simulink model "OpenLoopResponse"  (R2016a)
settings: Solver=VariableStepAuto  StartTime=0.0  StopTime=30  MaxStep=.005  RelTol=1e-3
libraries: simulink x1
settings Model: Creator=jordan  LastModifiedBy=jordan

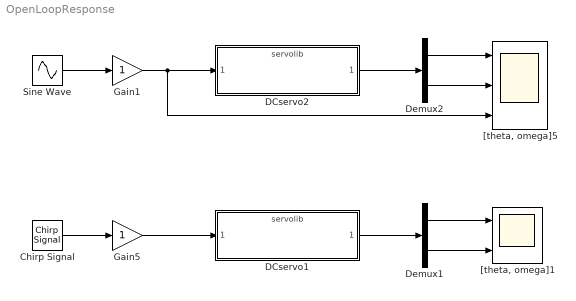
== system OpenLoopResponse ==
  Chirp Signal : simulink/Sources/Chirp Signal  f1=.01  T=120  f2=10
  DCservo1 : ModelReference  ModelNameDialog=servolib.slx  SimulationMode=Normal  ModelReferenceVersion=1.68
  DCservo2 : ModelReference  ModelNameDialog=servolib.slx  SimulationMode=Normal  ModelReferenceVersion=1.68
  Demux1 : Demux  Outputs=2
  Demux2 : Demux  Outputs=2
  Gain1 : Gain
  Gain5 : Gain
  Sine Wave : Sin  Frequency=10  SampleTime=0
  "[theta, omega]1" : Scope  NumInputPorts=2
  "[theta, omega]5" : Scope  NumInputPorts=3
  wires:
  DCservo2/1 -> Demux2/1
  Demux2/2 -> "[theta, omega]5"/2
  Demux2/1 -> "[theta, omega]5"/1
  Sine Wave/1 -> Gain1/1
  DCservo1/1 -> Demux1/1
  Demux1/2 -> "[theta, omega]1"/2
  Demux1/1 -> "[theta, omega]1"/1
  Chirp Signal/1 -> Gain5/1
  Gain5/1 -> DCservo1/1
  Gain1/1 -> "[theta, omega]5"/3, DCservo2/1
